simulink library "StewartControllers"  (Simulink 5.0)
values from neighbouring files (symbols this model uses):
  Ak = [-503.902978702 -9.65025283616 -1.61111571486 21.8428508942 -1.61111571545 -19.8533029484 -98379.7078721 -17056.4066886 3354.04339067 38923.095566 3416.49080336 -36645.6208433 ... (324 elements, 18x18)]    [StewartPlatformHinf.mat]
  Aw = [0 0 0 0 0 0 0 0 0 0 0 0 ... (36 elements, 6x6)]    [StewartPlatformHinf.mat]
  Bk = [503.902978702 9.65025283616 1.61111571486 -21.8428508942 1.61111571545 19.8533029484 59372.5849154 7558.20210451 916.385516522 -17079.290522 865.404764464 16116.257389 ... (216 elements, 18x12)]    [StewartPlatformHinf.mat]
  Bw = [316.227766017 0 0 0 0 0 0 316.227766017 0 0 0 0 ... (36 elements, 6x6)]    [StewartPlatformHinf.mat]
  Ck = [-1.000857122 0.000735828912456 0.000270297731214 -0.000282335636272 5.78181318491e-06 5.16610232519e-05 5.16611895171e-05 5.78186000017e-06 -0.000282335750675 0.000270298010313 0.000735828861314 -1.000857122 ... (108 elements, 6x18)]    [StewartPlatformHinf.mat]
  Cw = [316.227766017 0 0 0 0 0 0 316.227766017 0 0 0 0 ... (36 elements, 6x6)]    [StewartPlatformHinf.mat]
  D = inv(D)    [StewartMVController.m]    (also in StewartPlatformHinf.mat = [-0.999999982508 5.03947600575e-11 0.000132249034522 3.98267)
  Dk = [0 0 0 0 0 0 0 0 0 0 0 0 ... (72 elements, 6x12)]    [StewartPlatformHinf.mat]
  Dw = [20000000 0 0 0 0 0 0 20000000 0 0 0 0 ... (36 elements, 6x6)]    [StewartPlatformHinf.mat]
  Kd = 4.5e4    (= 45000)    [StewartPlatformSetup.m]
  Ki = 1e4    (= 10000)    [StewartPlatformSetup.m]
  Kp = 2e6    (= 2000000)    [StewartPlatformSetup.m]
  nomForces = [5184.22866413 5184.22866413 5184.22866413 5184.22866413 5184.22866413 5184.22866413]    [StewartPlatformHinf.mat]
undefined symbols (not defined in the file or in its folder): lower_leg_mass, top_mass, upper_leg_mass
libraries: StewartControllers x1
settings Model: Creator=jwendlan  LastModifiedBy=jwendlan

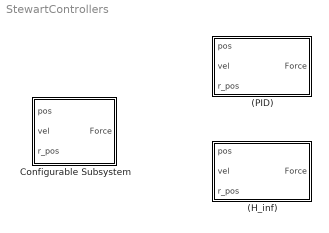
== system StewartControllers ==
  (H_inf) : Subsystem
  (PID) : Subsystem
  Configurable Subsystem : Subsystem  BlockChoice=(PID)
      settings: TemplateBlock=self  MemberBlocks=(H_inf),(PID)

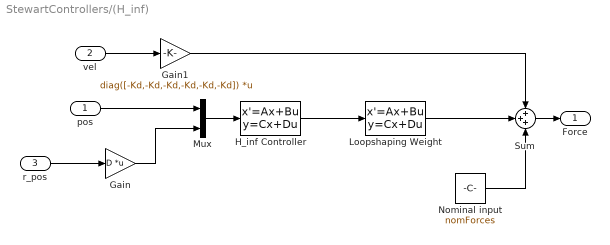
== system StewartControllers/(H_inf) ==
  pos : Inport
  vel : Inport  Port=2
  r_pos : Inport  Port=3
  Gain : Gain  Gain=D  Multiplication=Matrix(K*u)  SaturateOnIntegerOverflow=on
  Gain1 : Gain  Gain=diag([-Kd,-Kd,-Kd,-Kd,-Kd,-Kd])  Multiplication=Matrix(K*u)  SaturateOnIntegerOverflow=on
  H_inf Controller : StateSpace  A=Ak  B=Bk  C=Ck  D=Dk
  Loopshaping Weight : StateSpace  A=Aw  B=Bw  C=Cw  D=Dw
  Mux : Mux  Inputs=2
  Nominal input : Constant  Value=nomForces
  Sum : Sum  Inputs=+++  SaturateOnIntegerOverflow=on  InputSameDT=on
  Force : Outport
  wires:
  Gain1/1 -> Sum/1
  Loopshaping Weight/1 -> Sum/2
  Nominal input/1 -> Sum/3
  vel/1 -> Gain1/1
  Gain/1 -> Mux/2
  r_pos/1 -> Gain/1
  Sum/1 -> Force/1
  pos/1 -> Mux/1
  Mux/1 -> H_inf Controller/1
  H_inf Controller/1 -> Loopshaping Weight/1

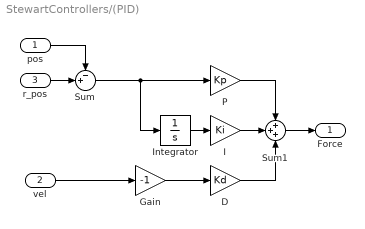
== system StewartControllers/(PID) ==
  pos : Inport
  vel : Inport  Port=2
  r_pos : Inport  Port=3
  D : Gain  Gain=Kd  SaturateOnIntegerOverflow=on
  Gain : Gain  Gain=-1  SaturateOnIntegerOverflow=on
  I : Gain  Gain=Ki  SaturateOnIntegerOverflow=on
  Integrator : Integrator  InitialCondition=(upper_leg_mass+lower_leg_mass+(top_mass*1.3/6))*9.81/Ki  ZeroCross=off
  P : Gain  Gain=Kp  SaturateOnIntegerOverflow=on
  Sum : Sum  Inputs=-+|  SaturateOnIntegerOverflow=on  InputSameDT=on
  Sum1 : Sum  Inputs=+++  SaturateOnIntegerOverflow=on  InputSameDT=on
  Force : Outport
  wires:
  Gain/1 -> D/1
  r_pos/1 -> Sum/2
  Sum1/1 -> Force/1
  pos/1 -> Sum/1
  D/1 -> Sum1/3
  vel/1 -> Gain/1
  Integrator/1 -> I/1
  P/1 -> Sum1/1
  I/1 -> Sum1/2
  Sum/1 -> Integrator/1, P/1

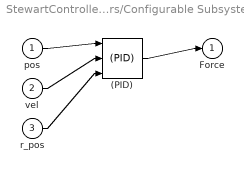
== system StewartControllers/Configurable Subsystem ==
  pos : Inport
  vel : Inport  Port=2
  r_pos : Inport  Port=3
  (PID) : StewartControllers/(PID)  SimViewingDevice=off  DataTypeOverride=UseLocalSettings  MinMaxOverflowLogging=UseLocalSettings
      settings: Permissions=ReadWrite  RTWFcnNameOpts=Auto  RTWFileNameOpts=Auto
  Force : Outport
  wires:
  pos/1 -> (PID)/1
  vel/1 -> (PID)/2
  r_pos/1 -> (PID)/3
  (PID)/1 -> Force/1
